simulink model "modelo"  (R2023a)
settings: Solver=VariableStepAuto  StartTime=0.0  StopTime=200  RelTol=1e-3
settings Model: Creator=ramir  LastModifiedBy=ramir
settings DataIOCC: ReturnWorkspaceOutputs=off  TimeSaveName=t

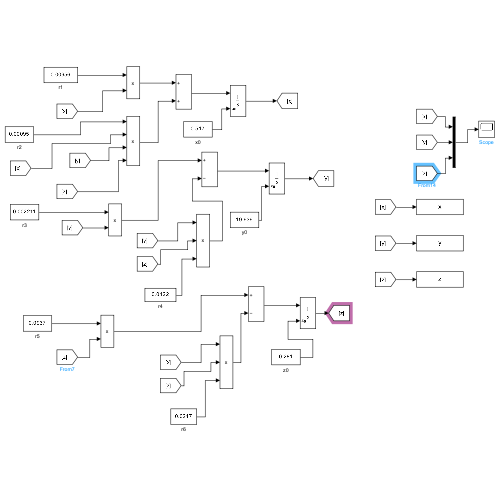
[thumbnail: Simulink's stored preview of the top-level diagram]
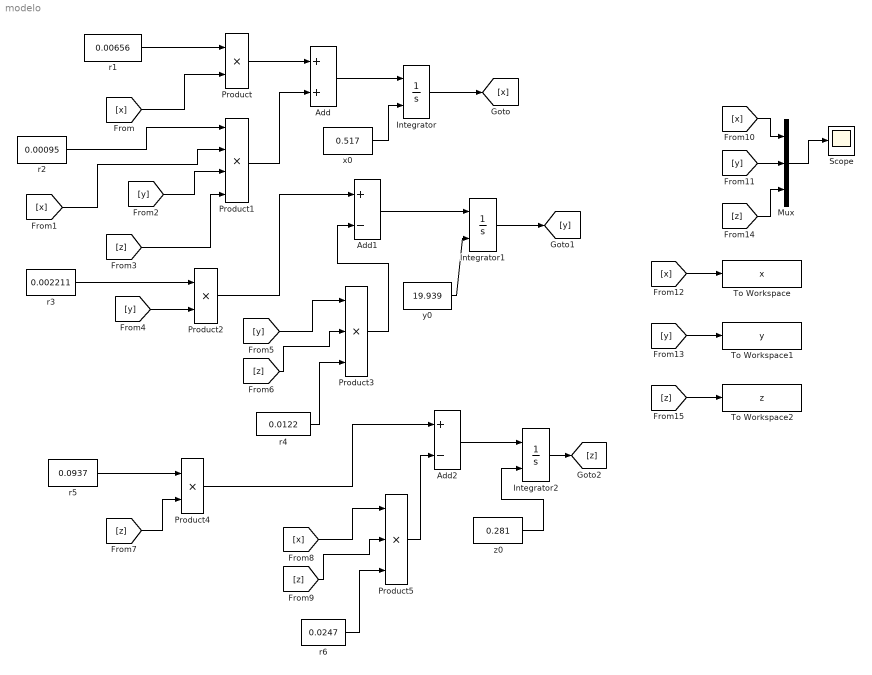
== system modelo ==
  Add : Sum
  Add1 : Sum  Inputs=+-
  Add2 : Sum  Inputs=+-
  Integrator : Integrator  InitialConditionSource=external
  Integrator1 : Integrator  InitialConditionSource=external
  Integrator2 : Integrator  InitialConditionSource=external
  Mux : Mux  Inputs=3
  Product : Product
  Product1 : Product  Inputs=4
  Product2 : Product
  Product3 : Product  Inputs=3
  Product4 : Product
  Product5 : Product  Inputs=3
  Scope : Scope
  To Workspace : ToWorkspace  VariableName=x  SampleTime=-1
  To Workspace1 : ToWorkspace  VariableName=y  SampleTime=-1
  To Workspace2 : ToWorkspace  VariableName=z  SampleTime=-1
  r1 : Constant  Value=0.00656
  r2 : Constant  Value=0.00095
  r3 : Constant  Value=0.002211
  r4 : Constant  Value=0.0122
  r5 : Constant  Value=0.0937
  r6 : Constant  Value=0.0247
  x0 : Constant  Value=0.517
  y0 : Constant  Value=19.939
  z0 : Constant  Value=0.281
  wires:
  r1/1 -> Product/1
  [x] -> Product/2
  Product/1 -> Add/1
  r2/1 -> Product1/1
  [x] -> Product1/2
  [y] -> Product1/3
  [z] -> Product1/4
  Product1/1 -> Add/2
  Add/1 -> Integrator/1
  x0/1 -> Integrator/2
  Integrator/1 -> [x]
  Product2/1 -> Add1/1
  r3/1 -> Product2/1
  [y] -> Product2/2
  [y] -> Product3/1
  [z] -> Product3/2
  r4/1 -> Product3/3
  Product3/1 -> Add1/2
  Add1/1 -> Integrator1/1
  y0/1 -> Integrator1/2
  Integrator1/1 -> [y]
  r5/1 -> Product4/1
  [z] -> Product4/2
  [x] -> Product5/1
  r6/1 -> Product5/3
  [z] -> Product5/2
  Product4/1 -> Add2/1
  Product5/1 -> Add2/2
  Add2/1 -> Integrator2/1
  z0/1 -> Integrator2/2
  Integrator2/1 -> [z]
  [y] -> To Workspace1/1
  [y] -> Mux/2
  Mux/1 -> Scope/1
  [x] -> Mux/1
  [x] -> To Workspace/1
  [z] -> Mux/3
  [z] -> To Workspace2/1
